simulink model "plant_block_swing_catch"  (R2013a)
settings: Solver=ode1  StartTime=0.0  StopTime=120  RelTol=1e-3
undefined symbols (not defined in the file or in its folder): magnitude
libraries: simulink x4
settings Model: SimulationMode=external  ExtModeTrigDuration=50000  Creator=Dro  LastModifiedBy=s4358762
settings DataIOCC: LimitDataPoints=off  SignalLoggingSaveFormat=ModelDataLogs  SignalLoggingName=sigsOut
settings OptimizationCC: ExpressionDepthLimit=2147483647  InitFltsAndDblsToZero=on
settings DebuggingCC: SaveWithParameterizedLinksMsg=none  SignalResolutionControl=TryResolveAllWithWarning  SolverPrmCheckMsg=none  MultiTaskDSMMsg=warning  MultiTaskCondExecSysMsg=none  FcnCallInpInsideContextMsg=UseLocalSettings  StrictBusMsg=None
settings RTWCC: SystemTargetFile=rtwin.tlc  TemplateMakefile=rtwin.tmf  Description=Real-Time Windows Target  ProcessScript=rtwin_make_rtw_hook  IncludeERTFirstTime=on
settings RTWinTargetCC: TargetFcnLib=ansi_tfl_tmw.mat  TargetLibSuffix=_rtwin.lib  TargetPreCompLibLocation=C:\Program Files\MATLAB\R2013a\toolbox\rtw\targets\rtwin\lib\win64  CodeReplacementLibrary=ANSI_C  ModelReferenceCompliant=off  CompOptLevelCompliant=off  RTWinDir=C:/PROGRA~1/MATLAB/R2013a/toolbox/rtw/targets/rtwin  TargetArch=win64

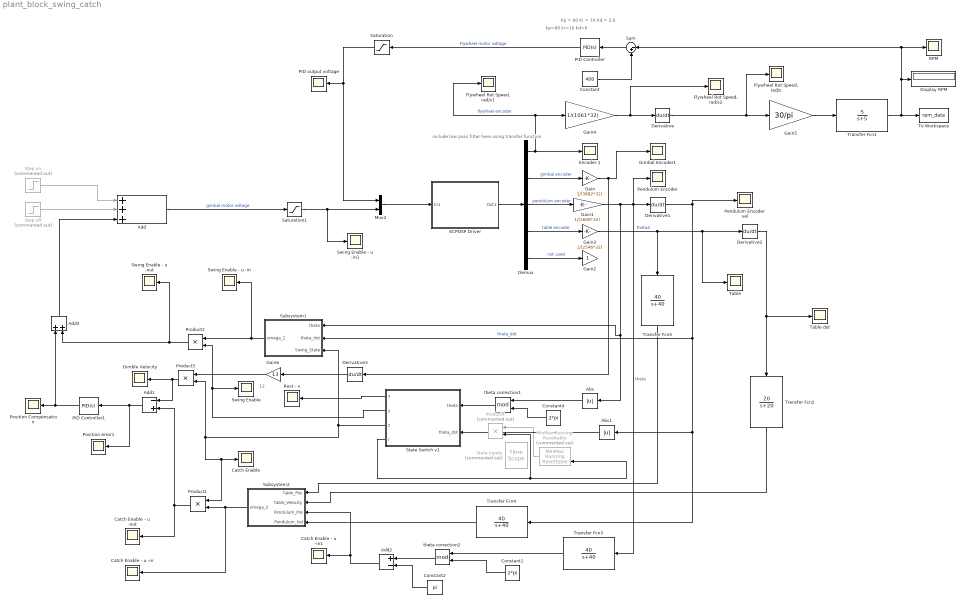
== system plant_block_swing_catch ==
  note: 12
  note: Kp = 60
      | Ki = 10
      | Kd = 2.6
  note: include low pass filter here
      | using transfer function
  note: kp=80
      | ki=16
      | kd=6
  Abs : Abs
  Abs1 : Abs
  Add : Sum  Inputs=+++
  Add1 : Sum  Inputs=-+
  Add2 : Sum  Inputs=+-
  Add3 : Sum
  Catch Enable : Scope
      settings: YMin=-10  YMax=10  SaveName=ScopeData12
  Catch Enable - u -in : Scope
      settings: YMin=-10  YMax=10  SaveName=ScopeData13
  Catch Enable - u -in1 : Scope
      settings: YMin=-10  YMax=10  SaveName=ScopeData26
  Catch Enable - u -out : Scope
      settings: YMin=-10  YMax=10  SaveName=ScopeData14
  Constant : Constant  Value=400
  Constant1 : Constant  Value=2*pi
  Constant2 : Constant  Value=pi
  Constant4 : Constant  Value=2*pi
  Demux : Demux  Outputs=5
  Derivative{,1..3} (4 alike) : Derivative
  Display RPM : Display
  ECPDSP Driver : Subsystem  mask{BaseAddr='0xC000', STime=0.008, TimeOutPer=500, HWAccess=on}
      mask prompts: BaseAddr "Base I/O Address"; STime "Sample Time (Sec)"; TimeOutPer "Timeout Period (500 ~ 2000)"; HWAccess "Hardware Access"
      mask Display: color('black');disp('ECPDSP Driver\n upto\n 4 Encs(ADC Channels)\n and 2 Dacs')
  Encoder 1 : Scope
      settings: YMin=1.5e+06  YMax=8.5e+06  SaveName=ScopeData3
  "Flywheel Rot Speed, rad/s" : Scope
  "Flywheel Rot Speed, rad/s1" : Scope
      settings: SaveName=ScopeData2
  "Flywheel Rot Speed, rad/s2" : Scope
      settings: SaveName=ScopeData4
  Gain : Gain  Gain=1/(3882*32)
  Gain1 : Gain  Gain=1/(2608*32)
  Gain2 : Gain
  Gain3 : Gain  Gain=1/(2546*32)
  Gain4 : Gain  Gain=1/(1061*32)
  Gain5 : Gain  Gain=30/pi
  Gain6 : Gain  Gain=13
  Gimbal Encoder1 : Scope
      settings: YMin=-0.25  YMax=3.25  SaveName=ScopeData9
  Gimble Velocity : Scope
      settings: YMin=-10  YMax=10  SaveName=ScopeData22
  MinMax Running Resettable : simulink/Math Operations/MinMax Running Resettable  Commented=on  Function=max  vinit=0.0
  Mux2 : Mux  Inputs=2
  PID Controller : simulink/Continuous/PID Controller  Controller=PID  TimeDomain=Continuous-time  SampleTime=1  IntegratorMethod=Forward Euler  FilterMethod=Forward Euler  Form=Parallel  P=60  I=10  D=2.6  N=100  InitialConditionSource=internal  InitialConditionForIntegrator=0  InitialConditionForFilter=0  ExternalReset=none  LimitOutput=off  UpperSaturationLimit=inf  LowerSaturationLimit=-inf  LinearizeAsGain=on  AntiWindupMode=none  Kb=1  TrackingMode=off  Kt=1  PParamMin=[]  PParamMax=[]  IParamMin=[]  IParamMax=[]  DParamMin=[]  DParamMax=[]  NParamMin=[]  NParamMax=[]  KbParamMin=[]  KbParamMax=[]  KtParamMin=[]  KtParamMax=[]  POutMin=[]  POutMax=[]  IOutMin=[]  IOutMax=[]  DOutMin=[]  DOutMax=[]  NOutMin=[]  NOutMax=[]  KbOutMin=[]  KbOutMax=[]  KtOutMin=[]  KtOutMax=[]  IntegratorOutMin=[]  IntegratorOutMax=[]  FilterOutMin=[]  FilterOutMax=[]  SumOutMin=[]  SumOutMax=[]  SumI1OutMin=[]  SumI1OutMax=[]  SumI2OutMin=[]  SumI2OutMax=[]  SumI3OutMin=[]  SumI3OutMax=[]  SumDOutMin=[]  SumDOutMax=[]  SaturationOutMin=[]  SaturationOutMax=[]  IntegratorContinuousStateAttributes=''  IntegratorStateMustResolveToSignalObject=off  IntegratorRTWStateStorageClass=Auto  FilterContinuousStateAttributes=''  FilterStateMustResolveToSignalObject=off  FilterRTWStateStorageClass=Auto
  PID Controller1 : simulink/Continuous/PID Controller  Controller=PID  TimeDomain=Continuous-time  SampleTime=1  IntegratorMethod=Forward Euler  FilterMethod=Forward Euler  Form=Parallel  P=120  I=5  D=0  N=100  InitialConditionSource=internal  InitialConditionForIntegrator=0  InitialConditionForFilter=0  ExternalReset=none  LimitOutput=off  UpperSaturationLimit=inf  LowerSaturationLimit=-inf  LinearizeAsGain=on  AntiWindupMode=none  Kb=1  TrackingMode=off  Kt=1  PParamMin=[]  PParamMax=[]  IParamMin=[]  IParamMax=[]  DParamMin=[]  DParamMax=[]  NParamMin=[]  NParamMax=[]  KbParamMin=[]  KbParamMax=[]  KtParamMin=[]  KtParamMax=[]  POutMin=[]  POutMax=[]  IOutMin=[]  IOutMax=[]  DOutMin=[]  DOutMax=[]  NOutMin=[]  NOutMax=[]  KbOutMin=[]  KbOutMax=[]  KtOutMin=[]  KtOutMax=[]  IntegratorOutMin=[]  IntegratorOutMax=[]  FilterOutMin=[]  FilterOutMax=[]  SumOutMin=[]  SumOutMax=[]  SumI1OutMin=[]  SumI1OutMax=[]  SumI2OutMin=[]  SumI2OutMax=[]  SumI3OutMin=[]  SumI3OutMax=[]  SumDOutMin=[]  SumDOutMax=[]  SaturationOutMin=[]  SaturationOutMax=[]  IntegratorContinuousStateAttributes=''  IntegratorStateMustResolveToSignalObject=off  IntegratorRTWStateStorageClass=Auto  FilterContinuousStateAttributes=''  FilterStateMustResolveToSignalObject=off  FilterRTWStateStorageClass=Auto
  PID output voltage : Scope
      settings: YMin=400  YMax=421  SaveName=ScopeData6
  Pendulum Encoder : Scope
      settings: YMin=-0.05  YMax=0.06  SaveName=ScopeData5
  Pendulum Encoder vel : Scope
      settings: YMin=-0.25  YMax=3.25  SaveName=ScopeData19
  Position Compensation : Scope
      settings: YMin=-10  YMax=10  SaveName=ScopeData20
  Position error1 : Scope
      settings: YMin=-10  YMax=10  SaveName=ScopeData21
  Product1 : Product
  Product2 : Product
  Product3 : Product
  Product4 : Product  Commented=on
  RPM : Scope
      settings: YMin=400  YMax=421
  Rest - x : Scope
      settings: YMin=-10  YMax=10  SaveName=ScopeData15
  Saturation : Saturate  UpperLimit=32000  LowerLimit=-32000
  Saturation1 : Saturate  UpperLimit=22000  LowerLimit=-22000
  State Inputs : TimeScope  Commented=on  NumInputPorts=2  DefaultConfigurationName=spbscopes.TimeScopeBlockCfg
      settings: CopyFcn=scopeextensions.ScopeBlock.callback(gcbh, 'onBlockCopy', gcbh);  DeleteFcn=scopeextensions.ScopeBlock.callback(gcbh, 'onBlockDelete');  PreSaveFcn=scopeextensions.ScopeBlock.callback(gcbh, 'onModelSave');  NameChangeFcn=scopeextensions.ScopeBlock.callback(gcbh, 'onBlockRename');  CloseFcn=scopeextensions.ScopeBlock.callback(gcbh, 'onBlockClose');  PreDeleteFcn=scopeextensions.ScopeBlock.callback(gcbh, 'onBlockPreDelete');
  State Switch v1 : Stateflow chart  TreatAsAtomicUnit=on
  Step off : Step  Commented=on  Time=30.15  After=-12000  SampleTime=0
  Step on : Step  Commented=on  Time=30  After=12000  SampleTime=0
  Subsystem1 : Subsystem
  Subsystem2 : Subsystem
  Sum : Sum  Inputs=|-+
  Swing Enable : Scope
      settings: YMin=-10  YMax=10  SaveName=ScopeData16
  Swing Enable - u -in : Scope
      settings: YMin=-10  YMax=10  SaveName=ScopeData17
  Swing Enable - u -in1 : Scope
      settings: YMin=-10  YMax=10  SaveName=ScopeData23
  Swing Enable - u -out : Scope
      settings: YMin=-10  YMax=10  SaveName=ScopeData18
  Table : Scope
      settings: YMin=-0.25  YMax=3.25  SaveName=ScopeData25
  Table dot : Scope
      settings: YMin=-0.25  YMax=3.25  SaveName=ScopeData24
  To Workspace : ToWorkspace  VariableName=rpm_data  SampleTime=-1  SaveFormat=Timeseries
  Transfer Fcn1 : TransferFcn  Numerator=[5]  Denominator=[1 5]
  Transfer Fcn2 : TransferFcn  Numerator=[20]  Denominator=[1 20]
  Transfer Fcn3 : TransferFcn  Numerator=[40]  Denominator=[1 40]
  Transfer Fcn4 : TransferFcn  Numerator=[40]  Denominator=[1 40]
  Transfer Fcn5 : TransferFcn  Numerator=[40]  Denominator=[1 40]
  theta correction1 : Math  Operator=mod  SaturateOnIntegerOverflow=on
  theta correction2 : Math  Operator=mod  SaturateOnIntegerOverflow=on
  wires:
  ECPDSP Driver/1(Out1) -> Demux/1
  Demux/1 -> Encoder 1/1, Gain4/1, "Flywheel Rot Speed, rad/s1"/1  "flywheel encoder"
  PID Controller/1 -> Saturation/1  "Flywheel motor voltage"
  Demux/2 -> Gain/1  "gimbal encoder"
  Demux/3 -> Gain1/1  "pendulum encoder"
  Demux/4 -> Gain3/1  "table encoder"
  Demux/5 -> Gain2/1  "not used"
  Gain4/1 -> "Flywheel Rot Speed, rad/s2"/1, Derivative/1
  Constant/1 -> Sum/2
  Sum/1 -> PID Controller/1
  Saturation/1 -> PID output voltage/1, Mux2/1
  Derivative/1 -> Gain5/1, "Flywheel Rot Speed, rad/s"/1
  Gain5/1 -> Transfer Fcn1/1
  Step off/1 -> Add/2
  Step on/1 -> Add/1
  Add/1 -> Saturation1/1  "gimbal motor voltage"
  Saturation1/1 -> Swing Enable - u -in1/1, Mux2/2
  Transfer Fcn1/1 -> To Workspace/1, Display RPM/1, RPM/1, Sum/1
  Derivative1/1 -> Transfer Fcn4/1, Abs1/1, Subsystem1/2(theta_dot), Pendulum Encoder vel/1  "theta_dot"
  Add3/1 -> Add/3
  State Switch v1/1(x) -> Rest - x/1
  theta correction1/1 -> State Switch v1/1(theta)
  Constant4/1 -> theta correction1/2
  Gain1/1 -> Abs/1, Subsystem1/1(theta), Transfer Fcn3/1, Pendulum Encoder/1, Derivative1/1  "theta"
  Subsystem1/1(omega_2) -> Product2/1, Swing Enable - u -in/1
  Gain3/1 -> Transfer Fcn5/1, Table/1, Derivative2/1  "theta4"
  Abs/1 -> theta correction1/1
  Subsystem2/1(omega_2) -> Catch Enable - u -in/1, Product1/2
  Product2/1 -> Add3/2, Swing Enable - u -out/1
  Derivative2/1 -> Table dot/1, Transfer Fcn2/1
  Gain/1 -> Derivative3/1, Gimbal Encoder1/1
  Add1/1 -> Position error1/1, PID Controller1/1
  PID Controller1/1 -> Add3/1, Position Compensation/1
  Derivative3/1 -> Gain6/1
  Product3/1 -> Add1/1, Gimble Velocity/1
  Product1/1 -> Catch Enable - u -out/1, Add1/2
  State Switch v1/3(z) -> Catch Enable/1, Product1/1, Product3/2, Subsystem1/3(Swing_State)
  Constant1/1 -> theta correction2/2
  theta correction2/1 -> Add2/1
  Constant2/1 -> Add2/2
  Add2/1 -> Catch Enable - u -in1/1, Subsystem2/3(Pendulum_Pos)
  Gain6/1 -> Product3/1
  Transfer Fcn2/1 -> Subsystem2/2(Table_Velocity)
  Transfer Fcn3/1 -> theta correction2/1
  Transfer Fcn4/1 -> Subsystem2/4(Pendulum_Vel)
  Transfer Fcn5/1 -> Subsystem2/1(Table_Pos)
  State Switch v1/4(r) -> Product4/2, MinMax Running Resettable/2
  MinMax Running Resettable/1 -> Product4/1
  Abs1/1 -> State Switch v1/2(theta_dot)
  State Switch v1/2(y) -> Swing Enable/1, Product2/2
  Mux2/1 -> ECPDSP Driver/1(In1)

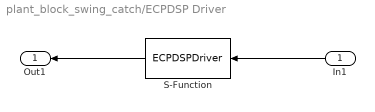
== system plant_block_swing_catch/ECPDSP Driver ==
  In1 : Inport
  S-Function : S-Function  FunctionName=ECPDSPDriver  Parameters=BaseAddr,STime,TimeOutPer,HWAccess  EnableBusSupport=off
  Out1 : Outport
  wires:
  In1/1 -> S-Function/1
  S-Function/1 -> Out1/1

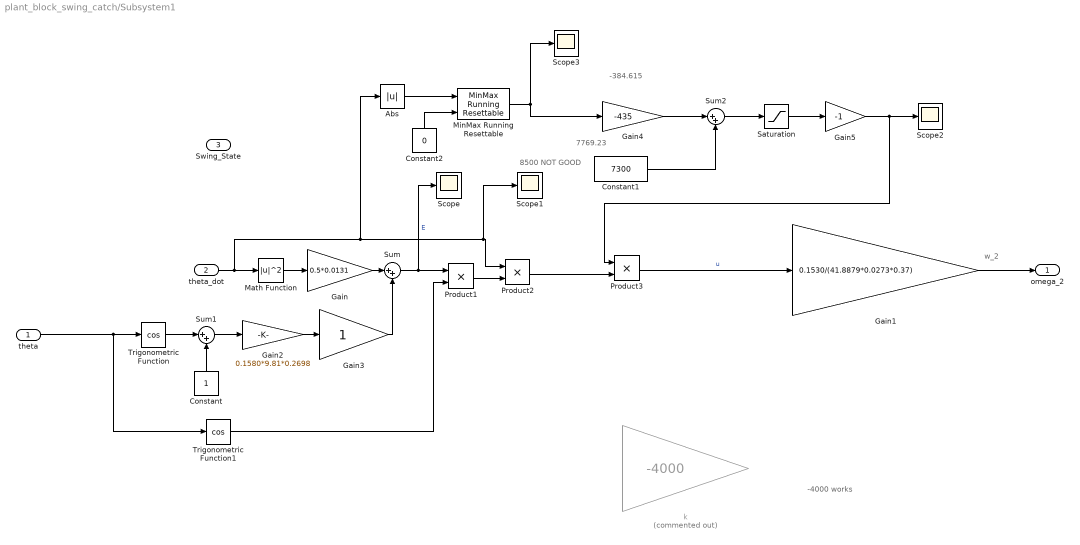
== system plant_block_swing_catch/Subsystem1 ==
  note: 8500 NOT GOOD
  note: 7769.23
  note: -384.615
  note: -4000 works
  note: w_2
  theta : Inport
  theta_dot : Inport  Port=2
  Swing_State : Inport  Port=3
  Abs : Abs
  Constant : Constant
  Constant1 : Constant  Value=7300
  Constant2 : Constant  Value=0
  Gain : Gain  Gain=0.5*0.0131
  Gain1 : Gain  Gain=0.1530/(41.8879*0.0273*0.37)
  Gain2 : Gain  Gain=0.1580*9.81*0.2698
  Gain3 : Gain
  Gain4 : Gain  Gain=-435
  Gain5 : Gain  Gain=-1
  Math Function : Math  Operator=magnitude^2  SaturateOnIntegerOverflow=on
  MinMax Running Resettable : simulink/Math Operations/MinMax Running Resettable  Function=max  vinit=0.0
  Product1 : Product
  Product2 : Product
  Product3 : Product
  Saturation : Saturate  UpperLimit=7300  LowerLimit=1400
  Scope{,1..3} (4 alike) : Scope
      Scope settings: YMin=-10  YMax=10  SaveName=ScopeData7
      Scope1 settings: YMin=-10  YMax=10  SaveName=ScopeData8
      Scope2 settings: YMin=-10  YMax=10  SaveName=ScopeData10
      Scope3 settings: YMin=-10  YMax=10  SaveName=ScopeData11
  Sum : Sum  Inputs=|++
  Sum1 : Sum  Inputs=|++
  Sum2 : Sum  Inputs=|++
  Trigonometric Function : Trigonometry  Operator=cos
  Trigonometric Function1 : Trigonometry  Operator=cos
  k : Gain  Commented=on  Gain=-4000
  omega_2 : Outport
  wires:
  theta_dot/1 -> Abs/1, Scope1/1, Product2/1, Math Function/1
  Math Function/1 -> Gain/1
  Gain/1 -> Sum/1
  Product3/1 -> Gain1/1  "u"
  Gain1/1 -> omega_2/1
  Trigonometric Function/1 -> Sum1/1
  Constant/1 -> Sum1/2
  Sum1/1 -> Gain2/1
  Gain2/1 -> Gain3/1
  Sum/1 -> Product1/1, Scope/1  "E"
  Trigonometric Function1/1 -> Product1/2
  Product1/1 -> Product2/2
  Product2/1 -> Product3/2
  theta/1 -> Trigonometric Function1/1, Trigonometric Function/1
  Gain3/1 -> Sum/2
  MinMax Running Resettable/1 -> Gain4/1, Scope3/1
  Gain4/1 -> Sum2/1
  Constant1/1 -> Sum2/2
  Sum2/1 -> Saturation/1
  Saturation/1 -> Gain5/1
  Gain5/1 -> Product3/1, Scope2/1
  Abs/1 -> MinMax Running Resettable/1
  Constant2/1 -> MinMax Running Resettable/2

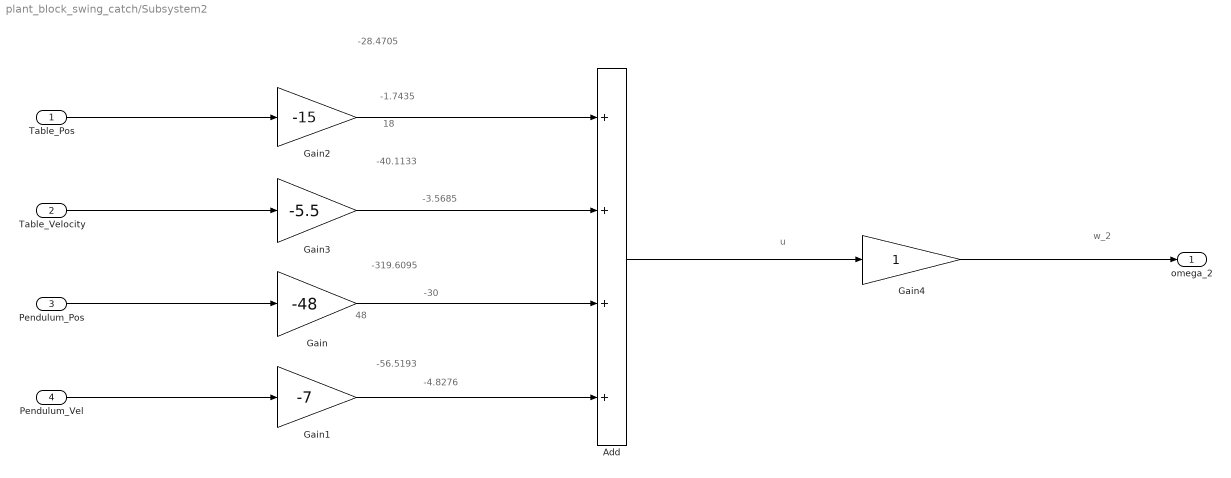
== system plant_block_swing_catch/Subsystem2 ==
  note: 18
  note: 48
  note: -4.8276
  note: -30
  note: -3.5685
  note: -1.7435
  note: -56.5193
  note: -319.6095
  note: -40.1133
  note: -28.4705
  note: w_2
  note: u
  Table_Pos : Inport
  Table_Velocity : Inport  Port=2
  Pendulum_Pos : Inport  Port=3
  Pendulum_Vel : Inport  Port=4
  Add : Sum  Inputs=++++
  Gain : Gain  Gain=-48
  Gain1 : Gain  Gain=-7
  Gain2 : Gain  Gain=-15
  Gain3 : Gain  Gain=-5.5
  Gain4 : Gain
  omega_2 : Outport
  wires:
  Gain2/1 -> Add/1
  Gain3/1 -> Add/2
  Table_Pos/1 -> Gain2/1
  Table_Velocity/1 -> Gain3/1
  Gain/1 -> Add/3
  Gain1/1 -> Add/4
  Pendulum_Pos/1 -> Gain/1
  Pendulum_Vel/1 -> Gain1/1
  Add/1 -> Gain4/1
  Gain4/1 -> omega_2/1

== stateflow chart plant_block_swing_catch/State Switch v1 ==
  state Swing
    entry:
    x = 0,
    y = 1,
    z = 0,
    r = 0;
  state Rest
    entry:
    x = 1,
    y = 0,
    z = 0;
    r = 0;
  state Catch
    entry:
    x = 0,
    y = 0,
    z = 1;
    r = 0;
  state ReSwing
    entry:
    x = 1,
    y = 0,
    z = 0;
    r = 1;
  (default) -> Rest
  Rest -> Swing : [theta > 0.12 & theta_dot > 0.12]
  ReSwing -> Swing : [theta_dot < 6]
  Swing -> Rest [order 2] : [theta < 0.12 & theta_dot < 0.12]
  Swing -> Catch [order 1] : [(3.14 - (3.14/8)) < theta & theta < (3.14 + (3.14/8))]
  Catch -> Swing [order 1] : [theta < (3.14 - (3.14/8)) | theta > (3.14 + (3.14/8))]
  Catch -> ReSwing [order 2] : [theta_dot > 12.5]
  data: x output; y output; z output; theta input; theta_dot input; r output
